simulink model "load_traj2"  (R2021a)
settings: Solver=ode45  StartTime=0.0  StopTime=inf  RelTol=1e-3  EnableMultiTasking=on
undefined symbols (not defined in the file or in its folder): f, RWS_Param
libraries: CarMaker4SL x31, instrumentlib x2, simulink x1
(part 1 of 2)
settings Model: ExtModeAutoUpdateStatusClock=off  Creator=fh  LastModifiedBy=ku347
settings SolverCC: AlgebraicLoopSolver=TrustRegion
settings DataIOCC: LimitDataPoints=on  SaveFormat=Array  SignalLoggingSaveFormat=ModelDataLogs  ReturnWorkspaceOutputs=off  SignalLoggingName=sigsOut
settings OptimizationCC: BooleanDataType=off  ExpressionDepthLimit=2147483647  InitFltsAndDblsToZero=on  LifeSpan=inf
settings DebuggingCC: SaveWithParameterizedLinksMsg=none  UnderspecifiedInitializationDetection=Classic  MergeDetectMultiDrivingBlocksExec=none  SignalResolutionControl=TryResolveAllWithWarning  MultiTaskDSMMsg=warning  MultiTaskCondExecSysMsg=none  FcnCallInpInsideContextMsg=warning  StateNameClashWarn=warning  SFUnexpectedBacktrackingDiag=warning  SFNoUnconditionalDefaultTransitionDiag=warning  SFMachineParentedDataDiag=warning  ArithmeticOperatorsInVariantConditions=warning
settings HardwareCC: ProdBitPerPointer=32  ProdBitPerSizeT=32  ProdBitPerPtrDiffT=32  ProdLargestAtomicFloat=None  ProdIntDivRoundTo=Undefined  ProdEndianess=Unspecified  ProdWordSize=32  ProdHWDeviceType=32-bit Generic  TargetUnknown=on
settings ModelReferenceCC: PropagateSignalLabelsOutOfModel=off
settings SFSimCC: SimUseLocalCustomCode=off  CustomCodeUndefinedFunction=UseInterfaceOnly
settings RTWCC: RTWUseLocalCustomCode=off
settings CodeAppCC: MaxIdLength=63  StateflowObjectComments=on
settings GRTTargetCC: TargetFcnLib=ansi_tfl_tmw.mat  TargetLangStandard=C89/C90 (ANSI)  CombineOutputUpdateFcns=off  GRTInterface=on
settings ConfigComp: CovMetricSettings=dw  CovSaveCumulativeToWorkspaceVar=on  CovSaveSingleToWorkspaceVar=on  CovExternalEMLEnable=off

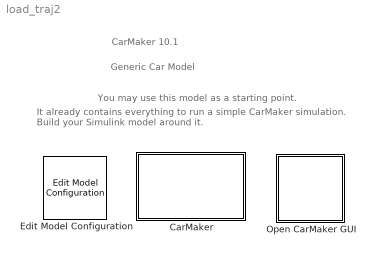
== system load_traj2 ==
  note: Generic Car Model
  note: You may use this model as a starting point.
  note: It already contains everything to run a simple CarMaker simulation.
      | Build your Simulink model around it.
  note: CarMaker 10.1
  CarMaker : Subsystem  TreatAsAtomicUnit=on
      mask Display: image(imread('CarMakerSys.png'));
  Edit Model Configuration : CarMaker4SL/Edit Model Configuration  SFunctionModules=''
  Open CarMaker GUI : Subsystem  LoadFcn=if ~length(which('cmself')), cmenv; end
      settings: OpenFcn=cmblockmagic('gui_fix_display'); CM_Simulink
      mask Display: image(imread('CarMakerGUI.png'));

== system load_traj2/CarMaker ==
  Bus Selector3 : BusSelector  OutputSignals=Speed[m/s]
  Bus Selector4 : BusSelector  OutputSignals=SteerAng[deg]
  CM_FIRST : Subsystem
  CM_LAST : Subsystem
      settings: PortSchema="{\"entries\":[{\"content\":{\"sides\":[{\"content\":{\"connectorIds\":[\"In1\"]},\"type\":\"ConnectorPlacement.EquallySpacedRectSide\",\"uuid\":\"564dcefc-e062-4aec-b6aa-852de86f2cab\"},{\"content\":{\"connectorIds\":[\"Out1\"],\"side\":\"RIGHT\"},\"type\":\"ConnectorPlacement.EquallySpacedRectSide\",\"uuid\":\"5b859068-20f3-4e40-9008-cd4c5872d7e0\"},{\"content\":{\"connectorIds\":[],\"side\":\"TOP\"},\"type\":\"ConnectorPlacement.EquallySpacedRectSide\",\"uuid\":\"172dd985-1669-44f7-9ac6-d507330b4777\"},{\"content\":{\"connectorIds\":[\"In2\"],\"side\":\"BOTTOM\"},\"type\":\"ConnectorPlacement.EquallySpacedRectSide\",\"uuid\":\"9436aa7f-11bf-4f1b-984f-027f2ad0c5a0\"}]},\"type\":\"ConnectorPlacement.EquallySpacedConnector\",\"uuid\":\"5160e0ba-90fd-48ff-84ef-d6e8c1c4e5f6\"}],\"packageUris\":[\"http://schema.mathworks.com/mf0/Connector/R2020b\"],\"version\":\"1.0\"}"
  DrivMan : Subsystem
  Ground : Ground
  IPG Vehicle : Subsystem  TreatAsAtomicUnit=on
  RWS : Subsystem  TreatAsAtomicUnit=on  SystemSampleTime=0.001
  Steering : Subsystem
  Terminator : Terminator
  VehicleControl : Subsystem
  Vehicle_Prameter : Subsystem
  Write CM Dict2 : CarMaker4SL/Write CM Dict  xname=Car.CRR.rz_ext  xsync=off
  Write CM Dict3 : CarMaker4SL/Write CM Dict  xname=Car.CRL.rz_ext  xsync=off
  wires:
  DrivMan/2(DrivMan.Out) -> VehicleControl/2(DrivMan.In)
  DrivMan/1(Sync_Out) -> VehicleControl/1(Sync_In)
  CM_FIRST/2(Env.Misc) -> DrivMan/2(Env.Misc)
  CM_FIRST/1(Sync_Out) -> DrivMan/1(Sync_In)
  CM_LAST/1(Sync_Out) -> Terminator/1
  Ground/1 -> CM_FIRST/1(Sync_In)
  IPG Vehicle/1(Sync_Out) -> CM_LAST/1(Sync_In)
  VehicleControl/1(Sync_Out) -> IPG Vehicle/1(Sync_In)
  VehicleControl/3(VhclCtrl.Steering) -> IPG Vehicle/3(VhclCtrl.Steering)
  VehicleControl/4(Vhcl.Wheel.In) -> IPG Vehicle/4(Vhcl.Wheel.In)
  VehicleControl/5(Vhcl.Misc) -> IPG Vehicle/5(Vhcl.Misc)
  VehicleControl/6(VhclCtrl.Brake) -> IPG Vehicle/6(VhclCtrl.Brake)
  VehicleControl/7(VhclCtrl.PT) -> IPG Vehicle/7(VhclCtrl.PT)
  VehicleControl/2(Vhcl.Model.Source) -> IPG Vehicle/2(Vhcl.Model.Source)
  RWS/1(Rear Road Wheel Angle (rad)) -> Write CM Dict2/1, Write CM Dict3/1  "y1"
  Bus Selector3/1 -> RWS/1(Vehicle_Speed [m/s])  "<Speed[m/s]>"
  Bus Selector4/1 -> RWS/2(Steering_Angle [deg])  "<SteerAng[deg]>"
  Vehicle_Prameter/1(Vehicle_Prameter) -> Bus Selector3/1
  Steering/1(Steering_Sensor) -> Bus Selector4/1
  VehicleControl/8(VhclCtrl.PT1) -> CM_LAST/2(VhclCtrl.PT1)

== system load_traj2/Open CarMaker GUI ==
  S-Function : S-Function  FunctionName=cm_gui  SFunctionDeploymentMode=off  EnableBusSupport=off

== system load_traj2/CarMaker/CM_FIRST ==
  Sync_In : Inport
  BusCreator1 : BusCreator  Inputs=8
  BusCreator2 : BusCreator  Inputs=6
  Demux1 : Demux  Outputs=14
      settings: DisplayOption=none
  Environment : S-Function  FunctionName=CM_Sfun  Parameters='Environment'  SFunctionDeploymentMode=off  EnableBusSupport=off
  IoIn : S-Function  FunctionName=CM_Sfun  Parameters='IoIn'  SFunctionDeploymentMode=off  EnableBusSupport=off
  Terminator : Terminator
  Sync_Out : Outport
  Env.Misc : Outport  Port=2
  wires:
  BusCreator2/1 -> Terminator/1  "IF Environment (in)"
  BusCreator1/1 -> Env.Misc/1
  Demux1/14 -> BusCreator2/6  "Env sRoad"
  Demux1/13 -> BusCreator2/5  "Env PoI_GCS Elev"
  Demux1/12 -> BusCreator2/4  "Env PoI_GCS Lat"
  Demux1/11 -> BusCreator2/3  "Env PoI_GCS Long"
  Demux1/10 -> BusCreator2/2  "Env Time"
  Demux1/9 -> BusCreator2/1  "Env yDay"
  Demux1/8 -> BusCreator1/8  "Env WindVel_tot z"
  Demux1/7 -> BusCreator1/7  "Env WindVel_tot y"
  Demux1/6 -> BusCreator1/6  "Env WindVel_tot x"
  Demux1/5 -> BusCreator1/5  "Env SolarRadiation"
  Demux1/4 -> BusCreator1/4  "Env AirHumidity"
  Demux1/3 -> BusCreator1/3  "Env AirPressure"
  Demux1/2 -> BusCreator1/2  "Env AirDensity"
  Demux1/1 -> BusCreator1/1  "Env Temperature"
  Environment/2 -> Demux1/1
  Environment/1 -> Sync_Out/1
  IoIn/1 -> Environment/1
  Sync_In/1 -> IoIn/1

== system load_traj2/CarMaker/CM_LAST ==
  Sync_In : Inport
  VhclCtrl.PT1 : Inport  Port=2
  CM_User : S-Function  FunctionName=CM_Sfun  Parameters='CM_User'  SFunctionDeploymentMode=off  EnableBusSupport=off
  Display : Display
  IoOut : S-Function  FunctionName=CM_Sfun  Parameters='IoOut'  SFunctionDeploymentMode=off  EnableBusSupport=off
  Mux : Mux  Inputs=6
  Read CM Dict : CarMaker4SL/Read CM Dict  xname=Sensor.Road.current.Path.tx  xsync=off  xstime=Continuous
  Read CM Dict1 : CarMaker4SL/Read CM Dict  xname=Sensor.Road.current.Path.ty  xsync=off  xstime=Continuous
  Read CM Dict2 : CarMaker4SL/Read CM Dict  xname=Time  xsync=off  xstime=Continuous
  Read CM Dict3 : CarMaker4SL/Read CM Dict  xname=Car.tx  xsync=off  xstime=Continuous
  Read CM Dict4 : CarMaker4SL/Read CM Dict  xname=Car.ty  xsync=off  xstime=Continuous
  tcpipsend : instrumentlib/TCP//IP Send  Host=127.0.0.1  Port=80  EnableBlockingMode=on  Timeout=30  ByteOrder=BigEndian  TransferDelay=on
  Sync_Out : Outport
  wires:
  IoOut/1 -> Sync_Out/1
  CM_User/1 -> IoOut/1
  Sync_In/1 -> CM_User/1
  Read CM Dict/1 -> Mux/4
  Mux/1 -> tcpipsend/1, Display/1
  Read CM Dict1/1 -> Mux/5
  VhclCtrl.PT1/1 -> Mux/6
  Read CM Dict2/1 -> Mux/1
  Read CM Dict3/1 -> Mux/2
  Read CM Dict4/1 -> Mux/3

== system load_traj2/CarMaker/DrivMan ==
  note: There's rarely a reason to override DrivMan signals.
      | Use the VehicleControl interface for this purpose.
  Sync_In : Inport
  Env.Misc : Inport  Port=2
  BusCreator : BusCreator  Inputs=17
  Demux : Demux  Outputs=17
      settings: DisplayOption=none
  DrivMan : S-Function  FunctionName=CM_Sfun  Parameters='DrivMan'  SFunctionDeploymentMode=off  EnableBusSupport=off
  Sync_Out : Outport
  DrivMan.Out : Outport  Port=2
  wires:
  Demux/17 -> BusCreator/17  "DrivMan Steering Trq"
  Demux/16 -> BusCreator/16  "DrivMan Steering AngAcc"
  Demux/15 -> BusCreator/15  "DrivMan Steering AngVel"
  Demux/14 -> BusCreator/14  "DrivMan Steering Ang"
  Demux/13 -> BusCreator/13  "DrivMan Gas"
  Demux/12 -> BusCreator/12  "DrivMan Clutch"
  Demux/11 -> BusCreator/11  "DrivMan BrakePark"
  Demux/10 -> BusCreator/10  "DrivMan Brake"
  Demux/9 -> BusCreator/9  "DrivMan GearNo"
  Demux/8 -> BusCreator/8  "DrivMan SelectorCtrl"
  Demux/7 -> BusCreator/7  "DrivMan UserSignal4"
  Demux/6 -> BusCreator/6  "DrivMan UserSignal3"
  Demux/5 -> BusCreator/5  "DrivMan UserSignal2"
  Demux/4 -> BusCreator/4  "DrivMan UserSignal1"
  Demux/3 -> BusCreator/3  "DrivMan UserSignal0"
  Demux/2 -> BusCreator/2  "DrivMan Key"
  Demux/1 -> BusCreator/1  "DrivMan SST"
  Env.Misc/1 -> DrivMan/2
  Sync_In/1 -> DrivMan/1
  DrivMan/1 -> Sync_Out/1
  BusCreator/1 -> DrivMan.Out/1
  DrivMan/2 -> Demux/1

== system load_traj2/CarMaker/IPG Vehicle ==
  Sync_In : Inport
  Vhcl.Model.Source : Inport  Port=2
  VhclCtrl.Steering : Inport  Port=3
  Vhcl.Wheel.In : Inport  Port=4
  Vhcl.Misc : Inport  Port=5
  VhclCtrl.Brake : Inport  Port=6
  VhclCtrl.PT : Inport  Port=7
  Brake : Subsystem
  CarAndTrailer : Subsystem
  PowerTrain : Subsystem
  Stop Simulation : Stop
  VehicleSource_BuiltIn : simulink/Logic and Bit Operations/Compare To Constant  relop=~=  const=1  OutDataTypeStr=boolean  ZeroCross=off
  Sync_Out : Outport
  wires:
  VhclCtrl.PT/1 -> PowerTrain/3(VhclCtrl.PT)
  Brake/1(Sync_Out) -> PowerTrain/1(Sync_In)
  CarAndTrailer/1(Sync_Out) -> Brake/1(Sync_In)
  CarAndTrailer/2(Brake.IF.In) -> Brake/2(Brake.IF.In)
  VhclCtrl.Brake/1 -> Brake/3(VhclCtrl.Brake)
  PowerTrain/1(Sync_Out) -> Sync_Out/1
  Vhcl.Misc/1 -> CarAndTrailer/4(Vhcl.Misc)
  Vhcl.Wheel.In/1 -> CarAndTrailer/3(Vhcl.Wheel.In)
  VhclCtrl.Steering/1 -> CarAndTrailer/2(VhclCtrl.Steering)
  Sync_In/1 -> CarAndTrailer/1(Sync_In)
  Vhcl.Model.Source/1 -> VehicleSource_BuiltIn/1
  VehicleSource_BuiltIn/1 -> Stop Simulation/1
  Brake/2(Vhcl.Wheel.PT) -> PowerTrain/2(Vhcl.Wheel.PT)

== system load_traj2/CarMaker/RWS ==
  Vehicle_Speed [m/s] : Inport
  Steering_Angle [deg] : Inport  Port=2
  DtoR : Gain  Gain=0.0174532925
  FWA_vs_RWA : Subsystem  TreatAsAtomicUnit=on  SystemSampleTime=0.001
  Frt_Wheel_Angle : Subsystem  TreatAsAtomicUnit=on  SystemSampleTime=0.001
  Product2 : Product
  Sign : Signum
  m/s to kph : Gain  Gain=3.6
  on/off : Gain
  Rear Road Wheel Angle (rad) : Outport
  wires:
  Frt_Wheel_Angle/1(Frt_Wheel_Angle [deg]) -> FWA_vs_RWA/2(Frt_Wheel_Angle [deg])  "Frt_Wheel_Angle [deg]"
  FWA_vs_RWA/1(Rear Wheel Angle [deg]) -> Product2/2  "Rear Wheel Angle [deg]"
  Steering_Angle [deg]/1 -> Sign/1, Frt_Wheel_Angle/1(SAS)
  Sign/1 -> Product2/1
  Product2/1 -> on/off/1
  m/s to kph/1 -> FWA_vs_RWA/1(Vehicle_Speed [kph])  "Vehicle_Speed_kph"
  Vehicle_Speed [m/s]/1 -> m/s to kph/1
  on/off/1 -> DtoR/1
  DtoR/1 -> Rear Road Wheel Angle (rad)/1

== system load_traj2/CarMaker/Steering ==
  Bus Creator : BusCreator  Inputs=7
  Ground : Ground
  Ground1 : Ground
  Read CM Dict1 : CarMaker4SL/Read CM Dict  xname=Steer.WhlTrq  xsync=off  xstime=Continuous
  Read CM Dict2 : CarMaker4SL/Read CM Dict  xname=Steer.WhlVel  xsync=off  xstime=Continuous
  Read CM Dict3 : CarMaker4SL/Read CM Dict  xname=Steer.AssistTrqCol  xsync=off  xstime=Continuous
  Read CM Dict4 : CarMaker4SL/Read CM Dict  xname=Steer.WhlAcc  xsync=off  xstime=Continuous
  Read CM Dict5 : CarMaker4SL/Read CM Dict  xname=Steer.WhlAng  xsync=off  xstime=Continuous
  Rename : Subsystem
  Rename1 : Subsystem
  Rename2 : Subsystem
  Rename3 : Subsystem
  UnitConversion1 : Subsystem  mask(UnitConversion){Selection=rad2deg}
      mask prompts: Selection "SelectUnitConversion"
      mask init:
      | switch Selection
      |     case 1 %rad2deg
      |         Offset = 0; Gain = 180/pi; Unit1 = 'rad'; Unit2 = 'deg';
      |     case 2 %deg2rad
      |         Offset = 0; Gain = pi/180; Unit1 = 'deg'; Unit2 = 'rad';
      |     case 3 %K2C
      |         Offset = -273.15; Gain = 1; Unit1 = 'K'; Unit2 = 'C';
      |     case 4 %C2K
      |         Offset = 273.15; Gain = 1; Unit1 = 'C'; Unit2 = 'K';
      |     case 5 %m/s2km/h
      |         Offset = 0; Gain = 3.6; Unit1 = 'm|s'; Unit2 = 'km|h';
      |     case 6 %km/h2m/s
      |         Offset = 0; Gain = 1/3.6; Unit1 = 'km|h'; Unit2 = 'm|s';
      |     case 7 %rad/s2rpm
      |         Offset = 0; Gain = 30/pi; Unit1 = 'rad|s'; Unit2 = 'rpm';
      |     case 8 %rpm2rad/s
      |         Offset = 0; Gain = pi/30; Unit1 = 'rpm'; Unit2 = 'rad|s';
      |     case 9 %none
      |         Offset = 0; Gain = 1; Unit1 = ''; Unit2 = '';
      |     case 10 %bar2Pa
      |         Offset = 0; Gain = 100000; Unit1 = 'bar'; Unit2 = 'Pa';
      |     case 11 %Pa2bar
      |         Offset = 0; Gain = 1/100000; Unit1 = 'Pa'; Unit2 = 'bar';
      |     case 12 %rad/s2Hz
      |         Offset = 0; Gain = 1/(2*pi); Unit1 = 'rad|s'; Unit2 = 'Hz';
      |     case 13 %Hz2rad/s
      |         Offset = 0; Gain = 2*pi; Unit1 = 'Hz'; Unit2 = 'rad|s';
      |     case 14 %psi2Pa
      |         Offset = 0; Gain = 6894.7567187; Unit1 = 'psi'; Unit2 = 'Pa';
      |     case 15 %Pa2psi
      |         Offset = 0; Gain = 0.000145; Unit1 = 'Pa'; Unit2 = 'psi';
      |     case 16   % %2[0..1]
      |         Offset = 0; Gain = 0.01; Unit1 = '%'; Unit2 = '0..1';
      |     case 17   % [0..1]2%
      |         Offset = 0; Gain = 100; Unit1 = '0..1'; Unit2 = '%';
      |     case 18	% Hz2rpm
      |         Offset = 0; Gain = 60 ; Unit1 = 'Hz'; Unit2 = 'rpm';
      |     case 19	% rpm2Hz
      |         Offset = 0; Gain = 0.0166667 ; Unit1 = 'rpm'; Unit2 = 'Hz';
      |     case 20	% Pa2hPa
      |         Offset = 0; Gain = 0.0100; Unit1 = 'Pa'; Unit2 = 'hPa';
      |     case 21  % hPa2Pa
      |         Offset = 0; Gain = 100; Unit1 = 'hPa'; Unit2 = 'Pa';
      |     case 22  % s2ms
      |         Offset = 0; Gain = 1000; Unit1 = 's'; Unit2 = 'ms';
      |     case 23	% ms2s
      |         Offset = 0; Gain = 0.001; Unit1 = 'ms'; Unit2 = 's';
      |     case 24	% K2F
      |         Offset = -494.741573; Gain = 1.797753; Unit1 = 'K'; Unit2 = 'F';
      |     case 25	% F2K
      |         Offset = 275.2; Gain = 0.55625 ; Unit1 = 'F'; Unit2 = 'K';
      |     otherwise
      |         Offset = 0; Gain = 1; Unit1 = 'Error'; Unit2 = 'Error';
      | end
      mask TypeOptions Selection: rad2deg | deg2rad | K2C | C2K | m/s2km/h | km/h2m/s | rad/s2rpm | rpm2rad/s | none | bar2Pa | Pa2bar | rad/s2Hz | Hz2rad/s | psi2Pa | Pa2psi | %2[0..1] | [0..1]2% | Hz2rpm | rpm2Hz | Pa2hPa | hPa2Pa | s2ms | ms2s | K2F | F2K
      mask Display:
      | port_label('input',1,['[', Unit1, ']'])
      | port_label('output',1, ['[', Unit2, ']'])
  UnitConversion2 : Subsystem  mask(UnitConversion){Selection=rad2deg}
      mask prompts: Selection "SelectUnitConversion"
      mask init: same as load_traj2/CarMaker/Steering/UnitConversion1
      mask TypeOptions Selection: rad2deg | deg2rad | K2C | C2K | m/s2km/h | km/h2m/s | rad/s2rpm | rpm2rad/s | none | bar2Pa | Pa2bar | rad/s2Hz | Hz2rad/s | psi2Pa | Pa2psi | %2[0..1] | [0..1]2% | Hz2rpm | rpm2Hz | Pa2hPa | hPa2Pa | s2ms | ms2s | K2F | F2K
      mask Display:
      | port_label('input',1,['[', Unit1, ']'])
      | port_label('output',1, ['[', Unit2, ']'])
  UnitConversion3 : Subsystem  mask(UnitConversion){Selection=rad2deg}
      mask prompts: Selection "SelectUnitConversion"
      mask init: same as load_traj2/CarMaker/Steering/UnitConversion1
      mask TypeOptions Selection: rad2deg | deg2rad | K2C | C2K | m/s2km/h | km/h2m/s | rad/s2rpm | rpm2rad/s | none | bar2Pa | Pa2bar | rad/s2Hz | Hz2rad/s | psi2Pa | Pa2psi | %2[0..1] | [0..1]2% | Hz2rpm | rpm2Hz | Pa2hPa | hPa2Pa | s2ms | ms2s | K2F | F2K
      mask Display:
      | port_label('input',1,['[', Unit1, ']'])
      | port_label('output',1, ['[', Unit2, ']'])
  Steering_Sensor : Outport
  wires:
  Rename/1(Out1) -> Bus Creator/4  "DrvSteerTrq[Nm]"
  UnitConversion1/1(Out) -> Bus Creator/2  "SteerVel[deg|s]"
  Read CM Dict5/1 -> UnitConversion3/1(In)  "SteerAng[rad]"
  Bus Creator/1 -> Steering_Sensor/1  "Steering_Sensor"
  UnitConversion2/1(Out) -> Bus Creator/3  "SteerAcc[deg|s^2]"
  Read CM Dict2/1 -> UnitConversion1/1(In)
  Read CM Dict4/1 -> UnitConversion2/1(In)
  Rename1/1(Out1) -> Bus Creator/5  "SteerAssistTrq[Nm]"
  Rename2/1(Out1) -> Bus Creator/6  "SteerSensTrq[Nm]"
  Rename3/1(Out1) -> Bus Creator/7  "SteerColTrq[Nm]"
  Read CM Dict1/1 -> Rename/1(In1)
  Read CM Dict3/1 -> Rename1/1(In1)
  Ground/1 -> Rename2/1(In1)
  Ground1/1 -> Rename3/1(In1)
  UnitConversion3/1(Out) -> Bus Creator/1  "SteerAng[deg]"

== system load_traj2/CarMaker/VehicleControl ==
  note: <Your model here>
  note: When implementing a vehicle control model,
      | be sure to add '-disablevehiclecontrol' to the command line arguments
      | in the CarMaker Model Configuration block.
      | Otherwise your model will possibly not see the original DrivMan signals
      | on its inputs, but those of a currently activated C-coded vehicle control model instead.
  Sync_In : Inport
  DrivMan.In : Inport  Port=2
  Bus Creator2 : BusCreator  Inputs=2
  CreateBus Vhcl.Misc : Subsystem
  CreateBus Vhcl.Wheel.In : Subsystem
  CreateBus VhclCtrl : Subsystem
  CreateBus VhclCtrl.PT : Subsystem
  CreateBus VhclCtrl.Steering : Subsystem
  Demux2 : Demux  Outputs=2
      settings: DisplayOption=none
  VehicleControl : S-Function  FunctionName=CM_Sfun  Parameters='VehicleControl'  SFunctionDeploymentMode=off  EnableBusSupport=off
  VehicleControlUpd : S-Function  FunctionName=CM_Sfun  Parameters='VehicleControlUpd'  SFunctionDeploymentMode=off  EnableBusSupport=off
  Sync_Out : Outport
  Vhcl.Model.Source : Outport  Port=2
  VhclCtrl.Steering : Outport  Port=3
  Vhcl.Wheel.In : Outport  Port=4
  Vhcl.Misc : Outport  Port=5
  VhclCtrl.Brake : Outport  Port=6
  VhclCtrl.PT : Outport  Port=7
  VhclCtrl.PT1 : Outport  Port=8
  wires:
  CreateBus VhclCtrl/1(Out) -> VehicleControlUpd/2
  VehicleControl/2 -> CreateBus VhclCtrl/1(In)
  VehicleControlUpd/2 -> Vhcl.Model.Source/1
  VehicleControlUpd/4 -> CreateBus Vhcl.Wheel.In/1(In1)
  VehicleControlUpd/5 -> CreateBus Vhcl.Misc/1(In1)
  VehicleControlUpd/6 -> Demux2/1
  VehicleControlUpd/7 -> CreateBus VhclCtrl.PT/1(In1)
  VehicleControlUpd/3 -> CreateBus VhclCtrl.Steering/1(In1)
  CreateBus Vhcl.Misc/1(Out1) -> Vhcl.Misc/1
  CreateBus Vhcl.Wheel.In/1(Out1) -> Vhcl.Wheel.In/1
  DrivMan.In/1 -> VehicleControl/2
  VehicleControl/1 -> VehicleControlUpd/1
  Sync_In/1 -> VehicleControl/1
  CreateBus VhclCtrl.PT/1(Out1) -> VhclCtrl.PT/1
  Bus Creator2/1 -> VhclCtrl.Brake/1
  CreateBus VhclCtrl.Steering/1(Out1) -> VhclCtrl.Steering/1
  VehicleControlUpd/1 -> Sync_Out/1
  Demux2/2 -> Bus Creator2/2  "VhclCtrl BrakePark"
  Demux2/1 -> Bus Creator2/1  "VhclCtrl Brake"
  CreateBus VhclCtrl/2(VhclCtrl.PT1) -> VhclCtrl.PT1/1

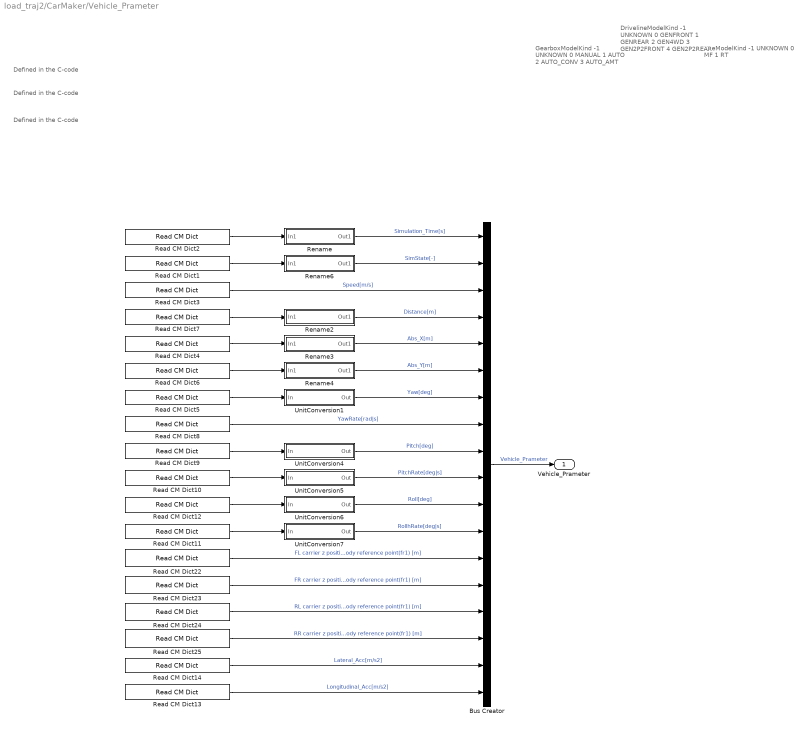
== system load_traj2/CarMaker/Vehicle_Prameter ==
  note: Defined in the C-code
  note: Defined in the C-code
  note: Defined in the C-code
  note: TireModelKind
      | -1 UNKNOWN
      | 0 MF
      | 1 RT
  note: DrivelineModelKind
      | -1 UNKNOWN
      | 0 GENFRONT
      | 1 GENREAR
      | 2 GEN4WD
      | 3 GEN2P2FRONT
      | 4 GEN2P2REAR
  note: GearboxModelKind
      | -1 UNKNOWN
      | 0 MANUAL
      | 1 AUTO
      | 2 AUTO_CONV
      | 3 AUTO_AMT
  Bus Creator : BusCreator  Inputs=18
  Read CM Dict1 : CarMaker4SL/Read CM Dict  xname=SC.State  xsync=off  xstime=Continuous
  Read CM Dict10 : CarMaker4SL/Read CM Dict  xname=Car.PitchAcc  xsync=off  xstime=Continuous
  Read CM Dict11 : CarMaker4SL/Read CM Dict  xname=Car.RollAcc  xsync=off  xstime=Continuous
  Read CM Dict12 : CarMaker4SL/Read CM Dict  xname=Car.Roll  xsync=off  xstime=Continuous
  Read CM Dict13 : CarMaker4SL/Read CM Dict  xname=Car.ax  xsync=off  xstime=Continuous
  Read CM Dict14 : CarMaker4SL/Read CM Dict  xname=Car.ay  xsync=off  xstime=Continuous
  Read CM Dict2 : CarMaker4SL/Read CM Dict  xname=Time  xsync=off  xstime=Continuous
  Read CM Dict22 : CarMaker4SL/Read CM Dict  xname=Car.CFL.tz  xsync=off  xstime=Continuous
  Read CM Dict23 : CarMaker4SL/Read CM Dict  xname=Car.CFR.tz  xsync=off  xstime=Continuous
  Read CM Dict24 : CarMaker4SL/Read CM Dict  xname=Car.CRL.tz  xsync=off  xstime=Continuous
  Read CM Dict25 : CarMaker4SL/Read CM Dict  xname=Car.CRR.tz  xsync=off  xstime=Continuous
  Read CM Dict3 : CarMaker4SL/Read CM Dict  xname=Car.v  xsync=off  xstime=Continuous
  Read CM Dict4 : CarMaker4SL/Read CM Dict  xname=Car.tx  xsync=off  xstime=Continuous
  Read CM Dict5 : CarMaker4SL/Read CM Dict  xname=Car.Yaw  xsync=off  xstime=Continuous
  Read CM Dict6 : CarMaker4SL/Read CM Dict  xname=Car.ty  xsync=off  xstime=Continuous
  Read CM Dict7 : CarMaker4SL/Read CM Dict  xname=Car.Distance  xsync=off  xstime=Continuous
  Read CM Dict8 : CarMaker4SL/Read CM Dict  xname=Car.YawRate  xsync=off  xstime=Continuous
  Read CM Dict9 : CarMaker4SL/Read CM Dict  xname=Car.Pitch  xsync=off  xstime=Continuous
  Rename : Subsystem
  Rename2 : Subsystem
  Rename3 : Subsystem
  Rename4 : Subsystem
  Rename6 : Subsystem
  UnitConversion1 : Subsystem  mask(UnitConversion){Selection=rad2deg}
      mask prompts: Selection "SelectUnitConversion"
      mask init: same as load_traj2/CarMaker/Steering/UnitConversion1
      mask TypeOptions Selection: rad2deg | deg2rad | K2C | C2K | m/s2km/h | km/h2m/s | rad/s2rpm | rpm2rad/s | none | bar2Pa | Pa2bar | rad/s2Hz | Hz2rad/s | psi2Pa | Pa2psi | %2[0..1] | [0..1]2% | Hz2rpm | rpm2Hz | Pa2hPa | hPa2Pa | s2ms | ms2s | K2F | F2K
      mask Display:
      | port_label('input',1,['[', Unit1, ']'])
      | port_label('output',1, ['[', Unit2, ']'])
  UnitConversion4 : Subsystem  mask(UnitConversion){Selection=rad2deg}
      mask prompts: Selection "SelectUnitConversion"
      mask init: same as load_traj2/CarMaker/Steering/UnitConversion1
      mask TypeOptions Selection: rad2deg | deg2rad | K2C | C2K | m/s2km/h | km/h2m/s | rad/s2rpm | rpm2rad/s | none | bar2Pa | Pa2bar | rad/s2Hz | Hz2rad/s | psi2Pa | Pa2psi | %2[0..1] | [0..1]2% | Hz2rpm | rpm2Hz | Pa2hPa | hPa2Pa | s2ms | ms2s | K2F | F2K
      mask Display:
      | port_label('input',1,['[', Unit1, ']'])
      | port_label('output',1, ['[', Unit2, ']'])
  UnitConversion5 : Subsystem  mask(UnitConversion){Selection=rad2deg}
      mask prompts: Selection "SelectUnitConversion"
      mask init: same as load_traj2/CarMaker/Steering/UnitConversion1
      mask TypeOptions Selection: rad2deg | deg2rad | K2C | C2K | m/s2km/h | km/h2m/s | rad/s2rpm | rpm2rad/s | none | bar2Pa | Pa2bar | rad/s2Hz | Hz2rad/s | psi2Pa | Pa2psi | %2[0..1] | [0..1]2% | Hz2rpm | rpm2Hz | Pa2hPa | hPa2Pa | s2ms | ms2s | K2F | F2K
      mask Display:
      | port_label('input',1,['[', Unit1, ']'])
      | port_label('output',1, ['[', Unit2, ']'])
  UnitConversion6 : Subsystem  mask(UnitConversion){Selection=rad2deg}
      mask prompts: Selection "SelectUnitConversion"
      mask init: same as load_traj2/CarMaker/Steering/UnitConversion1
      mask TypeOptions Selection: rad2deg | deg2rad | K2C | C2K | m/s2km/h | km/h2m/s | rad/s2rpm | rpm2rad/s | none | bar2Pa | Pa2bar | rad/s2Hz | Hz2rad/s | psi2Pa | Pa2psi | %2[0..1] | [0..1]2% | Hz2rpm | rpm2Hz | Pa2hPa | hPa2Pa | s2ms | ms2s | K2F | F2K
      mask Display:
      | port_label('input',1,['[', Unit1, ']'])
      | port_label('output',1, ['[', Unit2, ']'])
  UnitConversion7 : Subsystem  mask(UnitConversion){Selection=rad2deg}
      mask prompts: Selection "SelectUnitConversion"
      mask init: same as load_traj2/CarMaker/Steering/UnitConversion1
      mask TypeOptions Selection: rad2deg | deg2rad | K2C | C2K | m/s2km/h | km/h2m/s | rad/s2rpm | rpm2rad/s | none | bar2Pa | Pa2bar | rad/s2Hz | Hz2rad/s | psi2Pa | Pa2psi | %2[0..1] | [0..1]2% | Hz2rpm | rpm2Hz | Pa2hPa | hPa2Pa | s2ms | ms2s | K2F | F2K
      mask Display:
      | port_label('input',1,['[', Unit1, ']'])
      | port_label('output',1, ['[', Unit2, ']'])
  Vehicle_Prameter : Outport
  wires:
  Rename6/1(Out1) -> Bus Creator/2  "SimState[-]"
  Bus Creator/1 -> Vehicle_Prameter/1  "Vehicle_Prameter"
  Rename/1(Out1) -> Bus Creator/1  "Simulation_Time[s]"
  Read CM Dict3/1 -> Bus Creator/3  "Speed[m/s]"
  Rename2/1(Out1) -> Bus Creator/4  "Distance[m]"
  Rename3/1(Out1) -> Bus Creator/5  "Abs_X[m]"
  Rename4/1(Out1) -> Bus Creator/6  "Abs_Y[m]"
  UnitConversion1/1(Out) -> Bus Creator/7  "Yaw[deg]"
  Read CM Dict2/1 -> Rename/1(In1)
  Read CM Dict1/1 -> Rename6/1(In1)
  Read CM Dict5/1 -> UnitConversion1/1(In)
  Read CM Dict4/1 -> Rename3/1(In1)
  Read CM Dict6/1 -> Rename4/1(In1)
  Read CM Dict7/1 -> Rename2/1(In1)
  Read CM Dict8/1 -> Bus Creator/8  "YawRate[rad|s]"
  Read CM Dict10/1 -> UnitConversion5/1(In)
  Read CM Dict9/1 -> UnitConversion4/1(In)
  Read CM Dict12/1 -> UnitConversion6/1(In)
  Read CM Dict11/1 -> UnitConversion7/1(In)
  UnitConversion5/1(Out) -> Bus Creator/10  "PitchRate[deg|s]"
  UnitConversion4/1(Out) -> Bus Creator/9  "Pitch[deg]"
  UnitConversion6/1(Out) -> Bus Creator/11  "Roll[deg]"
  UnitConversion7/1(Out) -> Bus Creator/12  "RollhRate[deg|s]"
  Read CM Dict22/1 -> Bus Creator/13  "FL carrier z position from body reference point(fr1) [m]"
  Read CM Dict23/1 -> Bus Creator/14  "FR carrier z position from body reference point(fr1) [m]"
  Read CM Dict24/1 -> Bus Creator/15  "RL carrier z position from body reference point(fr1) [m]"
  Read CM Dict25/1 -> Bus Creator/16  "RR carrier z position from body reference point(fr1) [m]"
  Read CM Dict14/1 -> Bus Creator/17  "Lateral_Acc[m/s2]"
  Read CM Dict13/1 -> Bus Creator/18  "Longitudinal_Acc[m/s2]"

== system load_traj2/CarMaker/IPG Vehicle/Brake ==
  note: When replacing the entire braking system,
      | be sure to disable the IPG brake model by using the brake
      | model 'Model Manager off' in the vehicle GUI.
  note: <Your model here>
  Sync_In : Inport
  Brake.IF.In : Inport  Port=2
  VhclCtrl.Brake : Inport  Port=3
  Brake : S-Function  FunctionName=CM_Sfun  Parameters='Brake'  SFunctionDeploymentMode=off  EnableBusSupport=off
  BrakeUpd : S-Function  FunctionName=CM_Sfun  Parameters='BrakeUpd'  SFunctionDeploymentMode=off  EnableBusSupport=off
  BusCreator1 : BusCreator  Inputs=16
  CreateBus Vhcl.Wheel.PT : Subsystem
  Demux : Demux  Outputs=16
      settings: DisplayOption=none
  Sync_Out : Outport
  Vhcl.Wheel.PT : Outport  Port=2
  wires:
  Demux/16 -> BusCreator1/16  "Brake IF Trq_DriveSrc_trg d3"
  Demux/15 -> BusCreator1/15  "Brake IF Trq_DriveSrc_trg d2"
  Demux/14 -> BusCreator1/14  "Brake IF Trq_DriveSrc_trg d1"
  Demux/13 -> BusCreator1/13  "Brake IF Trq_DriveSrc_trg d0"
  Demux/12 -> BusCreator1/12  "Brake IF Trq_Reg_trg RR"
  Demux/11 -> BusCreator1/11  "Brake IF Trq_Reg_trg RL"
  Demux/10 -> BusCreator1/10  "Brake IF Trq_Reg_trg FR"
  Demux/9 -> BusCreator1/9  "Brake IF Trq_Reg_trg FL"
  Demux/8 -> BusCreator1/8  "Brake IF Trq_PB RR"
  Demux/7 -> BusCreator1/7  "Brake IF Trq_PB RL"
  Demux/6 -> BusCreator1/6  "Brake IF Trq_PB FR"
  Demux/5 -> BusCreator1/5  "Brake IF Trq_PB FL"
  Demux/4 -> BusCreator1/4  "Brake IF Trq_WB RR"
  Demux/3 -> BusCreator1/3  "Brake IF Trq_WB RL"
  Demux/2 -> BusCreator1/2  "Brake IF Trq_WB FR"
  Demux/1 -> BusCreator1/1  "Brake IF Trq_WB FL"
  Brake/2 -> Demux/1
  BusCreator1/1 -> BrakeUpd/2
  BrakeUpd/1 -> Sync_Out/1
  Brake/1 -> BrakeUpd/1  "Sync"
  Brake.IF.In/1 -> Brake/2
  VhclCtrl.Brake/1 -> Brake/3
  Sync_In/1 -> Brake/1
  BrakeUpd/2 -> CreateBus Vhcl.Wheel.PT/1(In)
  CreateBus Vhcl.Wheel.PT/1(Out) -> Vhcl.Wheel.PT/1

== system load_traj2/CarMaker/IPG Vehicle/CarAndTrailer ==
  Sync_In : Inport
  VhclCtrl.Steering : Inport  Port=2
  Vhcl.Wheel.In : Inport  Port=3
  Vhcl.Misc : Inport  Port=4
  CarAndTrailerUpd : Subsystem
  Forces : Subsystem
  Ground : Ground
  Kinematics : Subsystem
  Kinetics : Subsystem
  Steering : Subsystem
  Terminator : Terminator
  Terminator1 : Terminator
  Trailer : Subsystem
  Sync_Out : Outport
  Brake.IF.In : Outport  Port=2
  wires:
  Trailer/9(Car.Hitch.FrcTrq) -> CarAndTrailerUpd/9(Car.Hitch.FrcTrq)
  Trailer/8(Vhcl.Wheel.RR) -> CarAndTrailerUpd/8(Vhcl.Wheel.RR)
  Trailer/7(Vhcl.Wheel.RL) -> CarAndTrailerUpd/7(Vhcl.Wheel.RL)
  Trailer/6(Vhcl.Wheel.FR) -> CarAndTrailerUpd/6(Vhcl.Wheel.FR)
  Trailer/5(Vhcl.Wheel.FL) -> CarAndTrailerUpd/5(Vhcl.Wheel.FL)
  Trailer/4(Vhcl.PoI) -> CarAndTrailerUpd/4(Vhcl.PoI)
  Trailer/3(Vhcl.Motion) -> CarAndTrailerUpd/3(Vhcl.Motion)
  Trailer/2(Vhcl.Steering) -> CarAndTrailerUpd/2(Vhcl.Steering)
  Trailer/1(Sync_Out) -> CarAndTrailerUpd/1(Sync_In)
  CarAndTrailerUpd/2(Brake.IF.In) -> Brake.IF.In/1
  CarAndTrailerUpd/1(Sync_Out) -> Sync_Out/1
  Vhcl.Misc/1 -> Terminator1/1
  Vhcl.Wheel.In/1 -> Terminator/1
  Kinetics/6(WheelCarrier.Misc) -> Trailer/6(WheelCarrier.Misc)
  Kinetics/5(Car.Trq_T2W) -> Trailer/5(Car.Trq_T2W)
  Steering/2(Steer.IF) -> Kinematics/2(Steer.IF)
  Kinetics/4(Car.Fr1) -> Trailer/4(Car.Fr1)
  Kinetics/3(Car.Hitch) -> Trailer/3(Car.Hitch)
  Kinetics/2(Trailer.Load) -> Trailer/2(Trailer.Load)
  VhclCtrl.Steering/1 -> Steering/2(VhclCtrl.Steering)
  Sync_In/1 -> Steering/1(Sync_In)
  Steering/1(Sync_Out) -> Kinematics/1(Sync_In)
  Kinetics/1(Sync_Out) -> Trailer/1(Sync_In)
  Ground/1 -> CarAndTrailerUpd/10(Vhcl.Fr1A)
  Forces/11(FStabi_ext) -> Kinetics/11(FStabi_ext)
  Forces/10(FDamp_ext) -> Kinetics/10(FDamp_ext)
  Forces/9(FSpring_ext) -> Kinetics/9(FSpring_ext)
  Forces/8(TireRR_Out) -> Kinetics/8(TireRR.Out)
  Forces/7(TireRL_Out) -> Kinetics/7(TireRL.Out)
  Forces/6(TireFR_Out) -> Kinetics/6(TireFR.Out)
  Forces/5(TireFL_Out) -> Kinetics/5(TireFL.Out)
  Forces/4(Car.Load) -> Kinetics/4(Car.Load)
  Forces/2(Car.Virtual) -> Kinetics/2(Car.Virtual)
  Kinematics/6(lSpring) -> Forces/6(lSpring)
  Kinematics/7(vDamp) -> Forces/7(vDamp)
  Forces/3(Car.Aero) -> Kinetics/3(Car.Aero)
  Forces/1(Sync_Out) -> Kinetics/1(Sync_In)
  Kinematics/5(TireRR_In) -> Forces/5(TireRR_In)
  Kinematics/4(TireRL_In) -> Forces/4(TireRL_In)
  Kinematics/3(TireFR_In) -> Forces/3(TireFR_In)
  Kinematics/2(TireFL_In) -> Forces/2(TireFL_In)
  Kinematics/1(Sync_Out) -> Forces/1(Sync_In)
  Kinematics/8(lStabi) -> Forces/8(lStabi)
  Forces/12(FBuf_ext) -> Kinetics/12(FBuf_ext)
  Kinematics/9(lBuf) -> Forces/9(lBuf)

== system load_traj2/CarMaker/IPG Vehicle/PowerTrain ==
  note: When replacing the entire powertrain,
      | be sure to disable the IPG powertrain model by using the powertrain
      | model 'Model Manager off' in the vehicle GUI.
  note: <Your model here>
  Sync_In : Inport
  Vhcl.Wheel.PT : Inport  Port=2
  VhclCtrl.PT : Inport  Port=3
  BusCreator1 : BusCreator  Inputs=42
  Demux1 : Demux  Outputs=42
      settings: DisplayOption=none
  PowerTrain : S-Function  FunctionName=CM_Sfun  Parameters='PowerTrain'  SFunctionDeploymentMode=off  EnableBusSupport=off
  PowerTrainUpd : S-Function  FunctionName=CM_Sfun  Parameters='PowerTrainUpd'  SFunctionDeploymentMode=off  EnableBusSupport=off
  Sync_Out : Outport
  wires:
  BusCreator1/1 -> PowerTrainUpd/2
  Demux1/42 -> BusCreator1/42  "PT IF WRR Trq_BrakeReg_max"
  Demux1/41 -> BusCreator1/41  "PT IF WRR Trq_BrakeReg"
  Demux1/40 -> BusCreator1/40  "PT IF WRR Trq_Supp2WC"
  Demux1/39 -> BusCreator1/39  "PT IF WRR Trq_Drive"
  Demux1/38 -> BusCreator1/38  "PT IF WRR Trq_B2W"
  Demux1/37 -> BusCreator1/37  "PT IF WRR rotv"
  Demux1/36 -> BusCreator1/36  "PT IF WRR rot"
  Demux1/35 -> BusCreator1/35  "PT IF WRL Trq_BrakeReg_max"
  Demux1/34 -> BusCreator1/34  "PT IF WRL Trq_BrakeReg"
  Demux1/33 -> BusCreator1/33  "PT IF WRL Trq_Supp2WC"
  Demux1/32 -> BusCreator1/32  "PT IF WRL Trq_Drive"
  Demux1/31 -> BusCreator1/31  "PT IF WRL Trq_B2W"
  Demux1/30 -> BusCreator1/30  "PT IF WRL rotv"
  Demux1/29 -> BusCreator1/29  "PT IF WRL rot"
  Demux1/28 -> BusCreator1/28  "PT IF WFR Trq_BrakeReg_max"
  Demux1/27 -> BusCreator1/27  "PT IF WFR Trq_BrakeReg"
  Demux1/26 -> BusCreator1/26  "PT IF WFR Trq_Supp2WC"
  Demux1/25 -> BusCreator1/25  "PT IF WFR Trq_Drive"
  Demux1/24 -> BusCreator1/24  "PT IF WFR Trq_B2W"
  Demux1/23 -> BusCreator1/23  "PT IF WFR rotv"
  Demux1/22 -> BusCreator1/22  "PT IF WFR rot"
  Demux1/21 -> BusCreator1/21  "PT IF WFL Trq_BrakeReg_max"
  Demux1/20 -> BusCreator1/20  "PT IF WFL Trq_BrakeReg"
  Demux1/19 -> BusCreator1/19  "PT IF WFL Trq_Supp2WC"
  Demux1/18 -> BusCreator1/18  "PT IF WFL Trq_Drive"
  Demux1/17 -> BusCreator1/17  "PT IF WFL Trq_B2W"
  Demux1/16 -> BusCreator1/16  "PT IF WFL rotv"
  Demux1/15 -> BusCreator1/15  "PT IF WFL rot"
  Demux1/14 -> BusCreator1/14  "PT IF DL_iDiff_mean"
  Demux1/13 -> BusCreator1/13  "PT IF Trq_Supp2BdyEng y"
  Demux1/12 -> BusCreator1/12  "PT IF Trq_Supp2BdyEng x"
  Demux1/11 -> BusCreator1/11  "PT IF Trq_Supp2Bdy1B z"
  Demux1/10 -> BusCreator1/10  "PT IF Trq_Supp2Bdy1B y"
  Demux1/9 -> BusCreator1/9  "PT IF Trq_Supp2Bdy1B x"
  Demux1/8 -> BusCreator1/8  "PT IF Trq_Supp2Bdy1 z"
  Demux1/7 -> BusCreator1/7  "PT IF Trq_Supp2Bdy1 y"
  Demux1/6 -> BusCreator1/6  "PT IF Trq_Supp2Bdy1 x"
  Demux1/5 -> BusCreator1/5  "PT IF Engine_rotv"
  Demux1/4 -> BusCreator1/4  "PT IF GearNo"
  Demux1/3 -> BusCreator1/3  "PT IF OperationError"
  Demux1/2 -> BusCreator1/2  "PT IF OperationState"
  Demux1/1 -> BusCreator1/1  "PT IF Ignition"
  Sync_In/1 -> PowerTrain/1
  PowerTrain/2 -> Demux1/1
  PowerTrainUpd/1 -> Sync_Out/1
  PowerTrain/1 -> PowerTrainUpd/1  "Sync"
  VhclCtrl.PT/1 -> PowerTrain/3
  Vhcl.Wheel.PT/1 -> PowerTrain/2

== system load_traj2/CarMaker/RWS/FWA_vs_RWA ==
  Vehicle_Speed [kph] : Inport
  Frt_Wheel_Angle [deg] : Inport  Port=2
  Abs : Abs  SampleTime=0.001
  FWA_vs_RWA 2D Ratio : Lookup_n-D  NumberOfTableDimensions=1  BreakpointsForDimension1=RWS_Param.GEN1.THRESHOLD.AXIS_VEHICLE_SPEED_THRESHOLD  BreakpointsForDimension2=RWS_Param.GEN1.BASIC_RATIO.SAS_AXIS  Table=RWS_Param.GEN1.BASIC_RATIO.gf32_FWA_vs_RWA_1D_Ratio  ExtrapMethod=Clip  UseLastTableValue=on  SampleTime=0.001  RndMeth=Simplest  InputSameDT=on
  Product : Product
  Rear Wheel Angle [deg] : Outport
  wires:
  Vehicle_Speed [kph]/1 -> FWA_vs_RWA 2D Ratio/1
  Abs/1 -> Product/2
  Frt_Wheel_Angle [deg]/1 -> Abs/1
  FWA_vs_RWA 2D Ratio/1 -> Product/1
  Product/1 -> Rear Wheel Angle [deg]/1  "Target_Rear_Tire_Angle"

== system load_traj2/CarMaker/RWS/Frt_Wheel_Angle ==
  SAS : Inport
  Gain : Gain  Gain=1/14.7
  Frt_Wheel_Angle [deg] : Outport
  wires:
  SAS/1 -> Gain/1
  Gain/1 -> Frt_Wheel_Angle [deg]/1

== system load_traj2/CarMaker/Steering/Rename ==
  In1 : Inport
  Out1 : Outport
  wires:
  In1/1 -> Out1/1

== system load_traj2/CarMaker/Steering/Rename1 ==
  In1 : Inport
  Out1 : Outport
  wires:
  In1/1 -> Out1/1

== system load_traj2/CarMaker/Steering/Rename2 ==
  In1 : Inport
  Out1 : Outport
  wires:
  In1/1 -> Out1/1

== system load_traj2/CarMaker/Steering/Rename3 ==
  In1 : Inport
  Out1 : Outport
  wires:
  In1/1 -> Out1/1

== system load_traj2/CarMaker/Steering/UnitConversion1 ==
  In : Inport  Tag=inport
  Gain : Gain  Tag=u2_  Gain=Gain  SaturateOnIntegerOverflow=on  OutDataTypeStr=Inherit: Same as input  ParamDataTypeStr=Inherit: Same as input
  Offset : Constant  Tag=offset_  Value=Offset
  Sum : Sum  InputSameDT=on  SaturateOnIntegerOverflow=on  OutDataTypeStr=Inherit: Same as first input
  Out : Outport  Tag=outport
  wires:
  Sum/1 -> Out/1
  Gain/1 -> Sum/1
  Offset/1 -> Sum/2
  In/1 -> Gain/1

== system load_traj2/CarMaker/Steering/UnitConversion2 ==
  In : Inport  Tag=inport
  Gain : Gain  Tag=u2_  Gain=Gain  SaturateOnIntegerOverflow=on  OutDataTypeStr=Inherit: Same as input  ParamDataTypeStr=Inherit: Same as input
  Offset : Constant  Tag=offset_  Value=Offset
  Sum : Sum  InputSameDT=on  SaturateOnIntegerOverflow=on  OutDataTypeStr=Inherit: Same as first input
  Out : Outport  Tag=outport
  wires:
  In/1 -> Gain/1
  Offset/1 -> Sum/2
  Gain/1 -> Sum/1
  Sum/1 -> Out/1

== system load_traj2/CarMaker/Steering/UnitConversion3 ==
  In : Inport  Tag=inport
  Gain : Gain  Tag=u2_  Gain=Gain  SaturateOnIntegerOverflow=on  OutDataTypeStr=Inherit: Same as input  ParamDataTypeStr=Inherit: Same as input
  Offset : Constant  Tag=offset_  Value=Offset
  Sum : Sum  InputSameDT=on  SaturateOnIntegerOverflow=on  OutDataTypeStr=Inherit: Same as first input
  Out : Outport  Tag=outport
  wires:
  Sum/1 -> Out/1
  Gain/1 -> Sum/1
  Offset/1 -> Sum/2
  In/1 -> Gain/1

== system load_traj2/CarMaker/VehicleControl/CreateBus Vhcl.Misc ==
  In1 : Inport
  BusCreator : BusCreator  Inputs=11
  Demux : Demux  Outputs=11
      settings: DisplayOption=none
  Out1 : Outport
  wires:
  Demux/11 -> BusCreator/11  "Vhcl Wind_vel_0 z"
  Demux/10 -> BusCreator/10  "Vhcl Wind_vel_0 y"
  Demux/9 -> BusCreator/9  "Vhcl Wind_vel_0 x"
  Demux/8 -> BusCreator/8  "Vhcl Trq_DL2BdyEng y"
  Demux/7 -> BusCreator/7  "Vhcl Trq_DL2BdyEng x"
  Demux/6 -> BusCreator/6  "Vhcl Trq_DL2Bdy1B z"
  Demux/5 -> BusCreator/5  "Vhcl Trq_DL2Bdy1B y"
  Demux/4 -> BusCreator/4  "Vhcl Trq_DL2Bdy1B x"
  Demux/3 -> BusCreator/3  "Vhcl Trq_DL2Bdy1 z"
  Demux/2 -> BusCreator/2  "Vhcl Trq_DL2Bdy1 y"
  Demux/1 -> BusCreator/1  "Vhcl Trq_DL2Bdy1 x"
  In1/1 -> Demux/1
  BusCreator/1 -> Out1/1
